simulink model "BatteryModel"  (Simulink 8.8)
settings: Solver=ode1  StartTime=0.0  StopTime=Tend  FixedStep=1  RelTol=1e-3
values from neighbouring files (symbols this model uses):
  C1 = theta(3)    [run_model.m]
  Qnom = capacities(i)    [midterm.m]
  R0 = theta(1)    [run_model.m]
  R1 = theta(2)    [run_model.m]
  SOC0 = 1    [midterm.m]
  SOC_curve = Voc_data(:,1)    [run_model.m]    (also in run_validation_model.m)
  Voc_curve = Voc_data(:,2)    [run_model.m]    (also in run_validation_model.m)
libraries: simulink x1
settings Model: SuppressorTable=22 serialization::archive 11 0 3 0 0 0 0 0  Creator=Kramer  LastModifiedBy=Kramer
settings DataIOCC: LimitDataPoints=off  SaveFormat=Dataset  SignalLoggingSaveFormat=Dataset
settings OptimizationCC: LifeSpan=auto
settings DebuggingCC: UnderspecifiedInitializationDetection=Simplified  MergeDetectMultiDrivingBlocksExec=error  FcnCallInpInsideContextMsg=error  StateNameClashWarn=none  SFUnexpectedBacktrackingDiag=error  SFNoUnconditionalDefaultTransitionDiag=error  SFExecutionAtInitializationDiag=warning
settings HardwareCC: ProdBitPerPointer=64  ProdBitPerSizeT=64  ProdBitPerPtrDiffT=64  ProdLargestAtomicFloat=Float  ProdIntDivRoundTo=Zero  ProdEndianess=LittleEndian  ProdWordSize=64  ProdHWDeviceType=Intel->x86-64 (Windows64)
settings ModelReferenceCC: PropagateSignalLabelsOutOfModel=on
settings GRTTargetCC: TargetLangStandard=C99 (ISO)  GeneratePreprocessorConditionals=Use local settings  CombineOutputUpdateFcns=on  GRTInterface=off
settings ConfigComp: CovMetricSettings=dwe  CovHtmlReporting=off  CovSaveCumulativeToWorkspaceVar=off  CovSaveSingleToWorkspaceVar=off  CovExternalEMLEnable=on

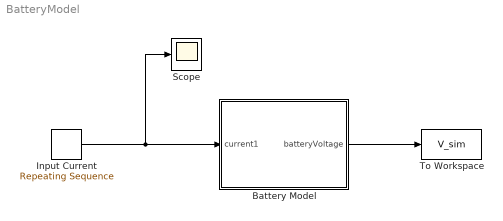
== system BatteryModel ==
  Battery Model : Subsystem
  Input Current : simulink/Sources/Repeating Sequence  rep_seq_t=t_data  rep_seq_y=I_data
  Scope : Scope
  To Workspace : ToWorkspace  VariableName=V_sim  SampleTime=-1
  wires:
  Input Current/1 -> Scope/1, Battery Model/1(current1)
  Battery Model/1(batteryVoltage) -> To Workspace/1

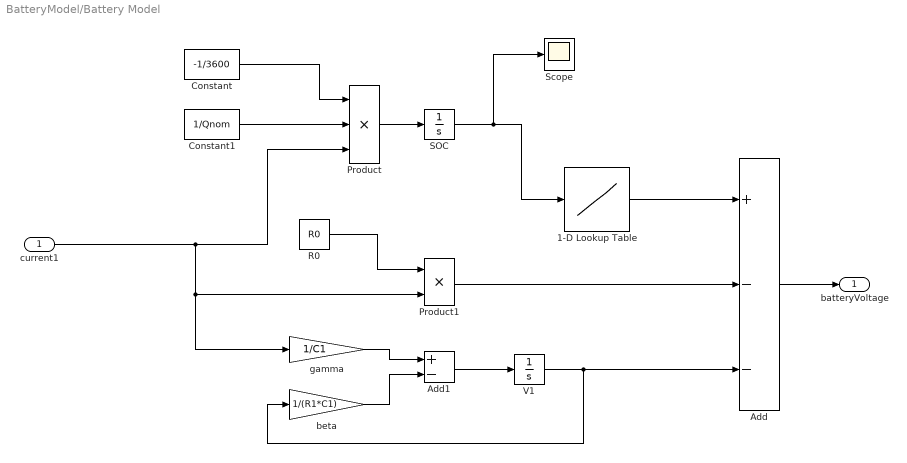
== system BatteryModel/Battery Model ==
  current1 : Inport
  1-D Lookup Table : Lookup_n-D  NumberOfTableDimensions=1  BreakpointsForDimension1=SOC_curve  Table=Voc_curve  InternalRulePriority=Speed  RndMeth=Simplest  InputSameDT=on
  Add : Sum  Inputs=+--
  Add1 : Sum  Inputs=+-
  Constant : Constant  Value=-1/3600
  Constant1 : Constant  Value=1/Qnom
  Product : Product  Inputs=3  RndMeth=Zero
  Product1 : Product  RndMeth=Zero
  R0 : Constant  Value=R0
  SOC : Integrator  InitialCondition=SOC0
  Scope : Scope
  V1 : Integrator
  beta : Gain  Gain=1/(R1*C1)
  gamma : Gain  Gain=1/C1
  batteryVoltage : Outport
  wires:
  Product/1 -> SOC/1
  Add/1 -> batteryVoltage/1
  Constant1/1 -> Product/2
  Add1/1 -> V1/1
  V1/1 -> beta/1, Add/3
  1-D Lookup Table/1 -> Add/1
  Constant/1 -> Product/1
  SOC/1 -> Scope/1, 1-D Lookup Table/1
  Product1/1 -> Add/2
  beta/1 -> Add1/2
  current1/1 -> Product1/2, gamma/1, Product/3
  gamma/1 -> Add1/1
  R0/1 -> Product1/1
